simulink model "chap7_4sim"  (Simulink 7.7)
settings: Solver=ode45  StartTime=0.0  StopTime=3  RelTol=1e-3
libraries: simulink x1
settings Model: Creator=liujk  LastModifiedBy=ljk  ExtModeTrigMode=oneshot  ExtModeArmWhenConnect=off
settings DataIOCC: Decimation=100  LimitDataPoints=off  SaveOutput=off  SaveTime=off  SignalLoggingName=sigsOut
settings OptimizationCC: BooleanDataType=off  ExpressionDepthLimit=128  InitFltsAndDblsToZero=on
settings DebuggingCC: SaveWithParameterizedLinksMsg=none  SignalResolutionControl=TryResolveAllWithWarning  SolverPrmCheckMsg=none  MultiTaskDSMMsg=warning  MultiTaskCondExecSysMsg=none  StrictBusMsg=None
settings HardwareCC: TargetUnknown=on
settings RTWCC: IncludeERTFirstTime=on
settings CodeAppCC: CustomSymbolStrType=$N$R$M_T
settings GRTTargetCC: TargetFcnLib=ansi_tfl_tmw.mat

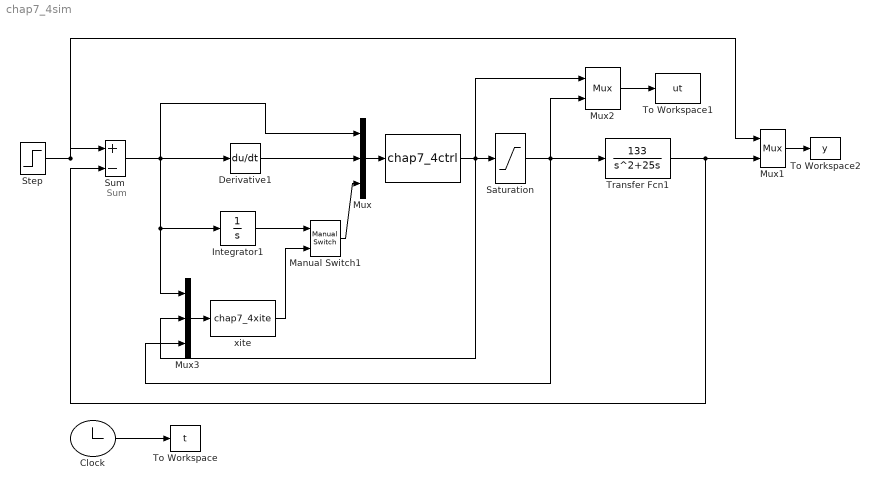
== system chap7_4sim ==
  note: Sum
  " " : S-Function  FunctionName=chap7_4ctrl  EnableBusSupport=off
  " xite" : S-Function  FunctionName=chap7_4xite  EnableBusSupport=off
  Clock : Clock
      settings: Decimation=10
  Derivative1 : Derivative
  Integrator1 : Integrator
  Manual Switch1 : simulink/Signal Routing/Manual Switch  SystemSampleTime=-1  sw=1  action=0  varsize=off
  Mux : Mux  Inputs=3
  Mux1 : Mux  Inputs=2
  Mux2 : Mux  Inputs=2
  Mux3 : Mux  Inputs=3
  Saturation : Saturate  UpperLimit=10  LowerLimit=0
  Step : Step  Time=0  After=10  SampleTime=0
  Sum : Sum  Inputs=|+-  SaturateOnIntegerOverflow=on  InputSameDT=on  OutDataTypeStr=Inherit: Same as first input
  To Workspace : ToWorkspace  VariableName=t  SampleTime=-1  SaveFormat=Array
  To Workspace1 : ToWorkspace  VariableName=ut  SampleTime=-1  SaveFormat=Array
  To Workspace2 : ToWorkspace  VariableName=y  SampleTime=-1  SaveFormat=Array
  Transfer Fcn1 : TransferFcn  Numerator=[133]  Denominator=[1 25 0]
  wires:
  Mux1/1 -> To Workspace2/1
  Transfer Fcn1/1 -> Mux1/2, Sum/2
  Saturation/1 -> Mux2/2, Transfer Fcn1/1, Mux3/3
  Step/1 -> Sum/1, Mux1/1
  Clock/1 -> To Workspace/1
  Sum/1 -> Mux/1, Mux3/1, Integrator1/1, Derivative1/1
  Mux/1 -> " "/1
  " "/1 -> Saturation/1, Mux2/1, Mux3/2
  Mux2/1 -> To Workspace1/1
  Derivative1/1 -> Mux/2
  Mux3/1 -> " xite"/1
  Integrator1/1 -> Manual Switch1/1
  " xite"/1 -> Manual Switch1/2
  Manual Switch1/1 -> Mux/3
